simulink model "ex1"  (Simulink 6.0)
settings: Solver=ode45  StartTime=0.0  StopTime=10.0  RelTol=1e-3
undefined symbols (not defined in the file or in its folder): functieg
settings Model: LastModifiedBy=student

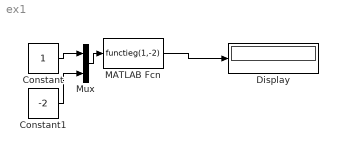
== system ex1 ==
  Constant : Constant
  Constant1 : Constant  Value=-2
  Display : Display
  MATLAB Fcn : MATLABFcn  MATLABFcn=functieg(1,-2)
  Mux : Mux  Inputs=2
  wires:
  Constant/1 -> Mux/1
  Constant1/1 -> Mux/2
  Mux/1 -> MATLAB Fcn/1
  MATLAB Fcn/1 -> Display/1
